simulink model "padTracking"  (R2014a)
settings: Solver=FixedStepDiscrete  StartTime=0.0  StopTime=inf  RelTol=1e-3
undefined symbols (not defined in the file or in its folder): fdesignblkfcn, gcbh
libraries: simulink x6, visionstatistics x3, visiontextngfix x2, embdlinuxlib x2
settings Model: SimulationMode=external  ExtModeTrigDuration=100  Creator=omcaree  LastModifiedBy=jsustare
settings OptimizationCC: OptimizeModelRefInitCode=on  LifeSpan=1
settings DebuggingCC: UnderspecifiedInitializationDetection=Classic  SolverPrmCheckMsg=none
settings HardwareCC: ProdLargestAtomicInteger=Long  ProdLargestAtomicFloat=Double  ProdEndianess=LittleEndian  ProdHWDeviceType=ARM Compatible->ARM Cortex
settings RTWCC: SystemTargetFile=realtime.tlc  GenerateMakefile=off  TemplateMakefile=realtime.tmf  Description=Run on Target Hardware  RTWVerbose=off  ProcessScript=realtime_make_rtw_hook
settings STFCustomTargetCC: TargetLibSuffix=.a  GenerateSampleERTMain=on  ConcurrentExecutionCompliant=off  GeneratePreprocessorConditionals=Use local settings  ERTCustomFileBanners=on  SupportNonInlinedSFcns=off  SupportVariableSizeSignals=on  MATLABClassNameForMDSCustomization=Simulink.SoftwareTarget.ERTCustomization  GRTInterface=off  SystemTargetFile=realtime.tlc
settings ERTTargetCC: CombineOutputUpdateFcns=off  SupportContinuousTime=on  SupportVariableSizeSignals=on  ExtMode=on  ExtModeMexArgs='169.254.0.31' 0 17725  ERTSrcFileBannerTemplate=realtime_code_template.cgt  ERTHdrFileBannerTemplate=realtime_code_template.cgt  ERTDataSrcFileTemplate=realtime_code_template.cgt  ERTDataHdrFileTemplate=realtime_code_template.cgt  ERTCustomFileTemplate=realtime_file_process.tlc

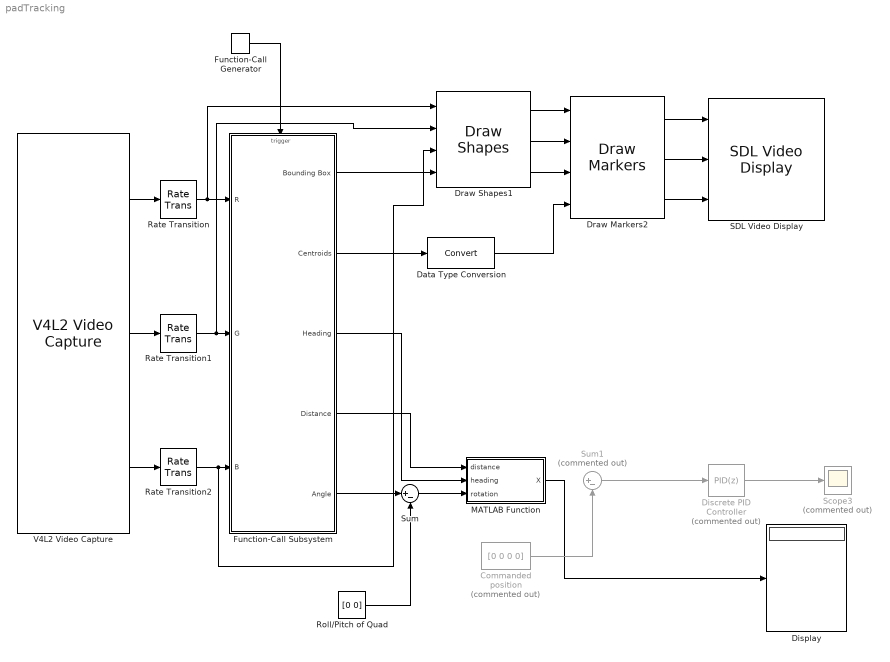
== system padTracking ==
  Commanded position : Constant  Commented=on  Value=[0 0 0 0]
  Data Type Conversion : DataTypeConversion
  Discrete PID Controller : simulink/Continuous/PID Controller  Commented=on  Controller=PID  TimeDomain=Discrete-time  SampleTime=-1  IntegratorMethod=Forward Euler  FilterMethod=Forward Euler  Form=Parallel  P=[1 1 1 1]  I=[0 0 0 0]  D=[0 0 0 0]  N=100  InitialConditionSource=internal  InitialConditionForIntegrator=0  InitialConditionForFilter=0  ExternalReset=none  LimitOutput=off  UpperSaturationLimit=inf  LowerSaturationLimit=-inf  LinearizeAsGain=off  AntiWindupMode=none  Kb=1  TrackingMode=off  Kt=1  PParamMin=[]  PParamMax=[]  IParamMin=[]  IParamMax=[]  DParamMin=[]  DParamMax=[]  NParamMin=[]  NParamMax=[]  KbParamMin=[]  KbParamMax=[]  KtParamMin=[]  KtParamMax=[]  POutMin=[]  POutMax=[]  IOutMin=[]  IOutMax=[]  DOutMin=[]  DOutMax=[]  NOutMin=[]  NOutMax=[]  KbOutMin=[]  KbOutMax=[]  KtOutMin=[]  KtOutMax=[]  IntegratorOutMin=[]  IntegratorOutMax=[]  FilterOutMin=[]  FilterOutMax=[]  SumOutMin=[]  SumOutMax=[]  SumI1OutMin=[]  SumI1OutMax=[]  SumI2OutMin=[]  SumI2OutMax=[]  SumI3OutMin=[]  SumI3OutMax=[]  SumDOutMin=[]  SumDOutMax=[]  SaturationOutMin=[]  SaturationOutMax=[]  IntegratorContinuousStateAttributes=''  IntegratorStateMustResolveToSignalObject=off  IntegratorRTWStateStorageClass=Auto  FilterContinuousStateAttributes=''  FilterStateMustResolveToSignalObject=off  FilterRTWStateStorageClass=Auto
  Display : Display
  Draw Markers2 : visiontextngfix/Draw Markers  shape=X-mark  size=3  fill=off  fillClrSource=Specify via dialog  display=User-specified value  intensity=200  color=[0 255 0; 255 0 0; 255 255 255]  opacity=0.6  viewport=Entire image  antialiasing=off  inType=Obsolete  imagePorts=Separate color signals  prodOutputMode=Binary point scaling  prodOutputWordLength=32  prodOutputFracLength=14  memoryMode=Specify word length  memoryWordLength=16  memoryFracLength=15  roundingMode=Floor  overflowMode=off
  Draw Shapes1 : visiontextngfix/Draw Shapes  shape=Rectangles  fill=off  lineWidth=1  fillClrSource=Specify via dialog  display=User-specified value  intensity=200  color=[255 0 0]  opacity=0.6  viewport=Entire image  antialiasing=off  inType=Obsolete  imagePorts=Separate color signals  prodOutputMode=Binary point scaling  prodOutputWordLength=32  prodOutputFracLength=14  memoryMode=Specify word length  memoryWordLength=16  memoryFracLength=15  roundingMode=Floor  overflowMode=off
  Function-Call Generator : simulink/Ports & Subsystems/Function-Call Generator  sample_time=3/30  numberOfIterations=1
  Function-Call Subsystem : Subsystem  TreatAsAtomicUnit=on
  MATLAB Function : MATLAB Function  TreatAsAtomicUnit=on
  Rate Transition : RateTransition  Deterministic=off
  Rate Transition1 : RateTransition  Deterministic=off
  Rate Transition2 : RateTransition  Deterministic=off
  Roll/Pitch of Quad : Constant  Value=[0 0]
  SDL Video Display : embdlinuxlib/SDL Video Display  pixelFormat=RGB  pixelOrder=Planar  rowMajor=on  blockPlatform=Raspberry Pi
  Scope3 : Scope  Commented=on
      settings: YMin=-0.05  YMax=0.65  SaveName=ScopeData3
  Sum : Sum  Inputs=|+-
  Sum1 : Sum  Commented=on  Inputs=|+-
  V4L2 Video Capture : embdlinuxlib/V4L2 Video Capture  m_devName='/dev/video0'  roi=[0, 0, 640, 480]  imSizeSelection=320x240  imSize=[640, 480]  pixelFormat=RGB  pixelOrder=Planar  sampleTime=1/30  simOutput=Colorbars  blockPlatform=Raspberry Pi
  wires:
  V4L2 Video Capture/3 -> Rate Transition2/1
  V4L2 Video Capture/1 -> Rate Transition/1
  V4L2 Video Capture/2 -> Rate Transition1/1
  Function-Call Generator/1 -> Function-Call Subsystem/Trigger
  Function-Call Subsystem/1(Bounding Box) -> Draw Shapes1/4
  Rate Transition/1 -> Draw Shapes1/1, Function-Call Subsystem/1(R)
  Rate Transition1/1 -> Draw Shapes1/2, Function-Call Subsystem/2(G)
  Rate Transition2/1 -> Draw Shapes1/3, Function-Call Subsystem/3(B)
  Data Type Conversion/1 -> Draw Markers2/4
  Function-Call Subsystem/2(Centroids) -> Data Type Conversion/1
  Function-Call Subsystem/4("Distance ") -> MATLAB Function/1(distance)
  Function-Call Subsystem/5(Angle) -> Sum/1
  Sum/1 -> MATLAB Function/3(rotation)
  Roll/Pitch of Quad/1 -> Sum/2
  MATLAB Function/1(X) -> Display/1
  Commanded position/1 -> Sum1/2
  Sum1/1 -> Discrete PID Controller/1
  Discrete PID Controller/1 -> Scope3/1
  Draw Markers2/2 -> SDL Video Display/2
  Draw Markers2/3 -> SDL Video Display/3
  Draw Markers2/1 -> SDL Video Display/1
  Draw Shapes1/3 -> Draw Markers2/3
  Draw Shapes1/2 -> Draw Markers2/2
  Draw Shapes1/1 -> Draw Markers2/1
  Function-Call Subsystem/3(Heading) -> MATLAB Function/2(heading)

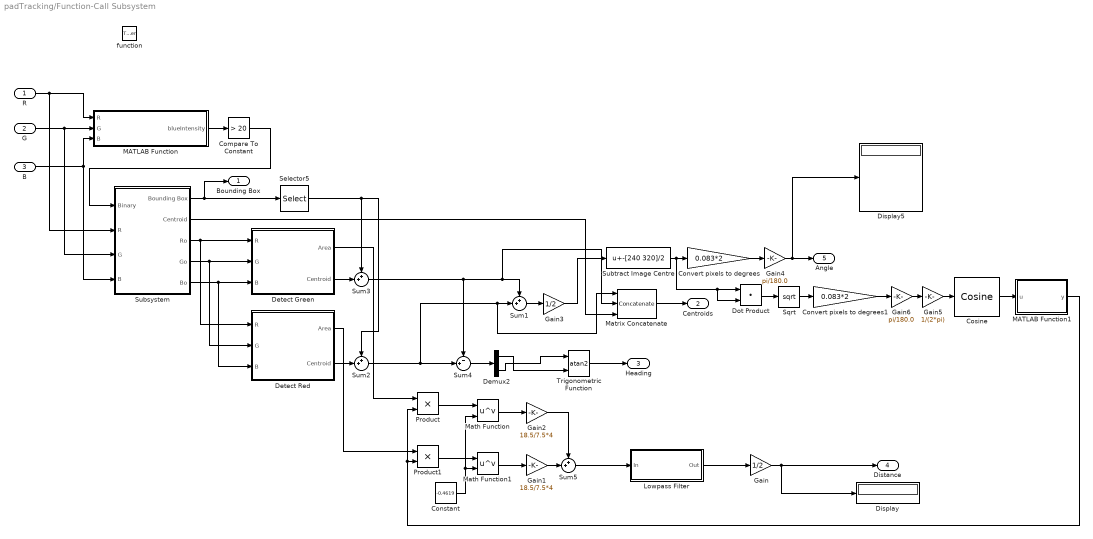
== system padTracking/Function-Call Subsystem ==
  R : Inport
  G : Inport  Port=2
  B : Inport  Port=3
  function : TriggerPort  TriggerType=function-call
  Compare To Constant : simulink/Logic and Bit Operations/Compare To Constant  relop=>  const=20  OutDataTypeStr=boolean
  Constant : Constant  Value=-0.4619
  Convert pixels to degrees : Gain  Gain=0.083*2
  Convert pixels to degrees1 : Gain  Gain=0.083*2
  Cosine : simulink/Lookup Tables/Cosine  Formula=cos(2*pi*u)  NumDataPoints=(2^5)+1  OutputWordLength=16  InternalRulePriority=Speed
  Demux2 : Demux  Outputs=2
  Detect Green : Subsystem
  Detect Red : Subsystem
  Display : Display
  Display5 : Display
  Dot Product : DotProduct  InputSameDT=on  OutDataTypeStr=Inherit: Inherit via internal rule
  Gain : Gain  Gain=1/2
  Gain1 : Gain  Gain=18.5/7.5*4
  Gain2 : Gain  Gain=18.5/7.5*4
  Gain3 : Gain  Gain=1/2
  Gain4 : Gain  Gain=pi/180.0
  Gain5 : Gain  Gain=1/(2*pi)
  Gain6 : Gain  Gain=pi/180.0
  Lowpass Filter : Subsystem  DialogController=fdesignblkfcn  InitFcn=fdesignblkfcn(gcbh, {'InitFcn'});  mask(Lowpass Filter){}
      mask help: Design a lowpass filter
      settings: CopyFcn=fdesignblkfcn(gcbh, {'CopyFcn'});
      mask Help: helpview(mapfilelocation('dsp'), 'dsplowpassfilter');
      mask Display: disp('Lowpass')
  MATLAB Function : MATLAB Function  TreatAsAtomicUnit=on
  MATLAB Function1 : MATLAB Function  TreatAsAtomicUnit=on
  Math Function : Math  Operator=pow  SaturateOnIntegerOverflow=on
  Math Function1 : Math  Operator=pow  SaturateOnIntegerOverflow=on
  Matrix Concatenate : Concatenate  NumInputs=3  Mode=Multidimensional array
  Product : Product
  Product1 : Product
  Selector5 : Selector  InputPortWidth=4  Indices=[1 2]
  Sqrt : Sqrt  SaturateOnIntegerOverflow=on
  Subsystem : Subsystem
  Subtract Image Centre : Bias  Bias=-[240 320]/2
  Sum{1..3,5} (4 alike) : Sum  Inputs=++|
  Sum4 : Sum  Inputs=-+|
  Trigonometric Function : Trigonometry  Operator=atan2
  Bounding Box : Outport
  Centroids : Outport  Port=2
  Heading : Outport  Port=3
  "Distance " : Outport  Port=4
  Angle : Outport  Port=5
  wires:
  G/1 -> MATLAB Function/2(G), Subsystem/3(G)
  R/1 -> MATLAB Function/1(R), Subsystem/2(R)
  MATLAB Function/1(blueIntensity) -> Compare To Constant/1
  Compare To Constant/1 -> Subsystem/1(Binary)
  B/1 -> Subsystem/4(B), MATLAB Function/3(B)
  Selector5/1 -> Sum3/1, Sum2/1
  Sum2/1 -> Matrix Concatenate/1, Sum1/2, Sum4/2
  Sum4/1 -> Demux2/1
  Math Function1/1 -> Gain1/1
  Math Function/1 -> Gain2/1
  Constant/1 -> Math Function/2, Math Function1/2
  Demux2/2 -> Trigonometric Function/1
  Demux2/1 -> Trigonometric Function/2
  Detect Green/1(Area) -> Product/1
  Detect Green/2(Centroid) -> Sum3/2
  Detect Red/1(Area) -> Product1/1
  Detect Red/2(Centroid) -> Sum2/2
  Subsystem/3(Ro) -> Detect Red/1(R), Detect Green/1(R)
  Subsystem/5(Bo) -> Detect Red/3(B), Detect Green/3(B)
  Subsystem/4(Go) -> Detect Red/2(G), Detect Green/2(G)
  Subsystem/1(Bounding Box) -> Selector5/1, Bounding Box/1
  Trigonometric Function/1 -> Heading/1
  Gain/1 -> "Distance "/1, Display/1
  Sum1/1 -> Gain3/1
  Gain3/1 -> Subtract Image Centre/1
  Sum3/1 -> Matrix Concatenate/2, Sum1/1, Sum4/1
  Gain2/1 -> Sum5/1
  Gain1/1 -> Sum5/2
  Subtract Image Centre/1 -> Dot Product/2, Dot Product/1, Convert pixels to degrees/1
  Convert pixels to degrees/1 -> Gain4/1
  Gain4/1 -> Display5/1, Angle/1
  Matrix Concatenate/1 -> Centroids/1
  Subsystem/2(Centroid) -> Matrix Concatenate/3
  Lowpass Filter/1(Out) -> Gain/1
  Gain5/1 -> Cosine/1
  Convert pixels to degrees1/1 -> Gain6/1
  Gain6/1 -> Gain5/1
  Dot Product/1 -> Sqrt/1
  Sqrt/1 -> Convert pixels to degrees1/1
  Sum5/1 -> Lowpass Filter/1(In)
  Product/1 -> Math Function/1
  Product1/1 -> Math Function1/1
  MATLAB Function1/1(y) -> Product1/2, Product/2
  Cosine/1 -> MATLAB Function1/1(u)

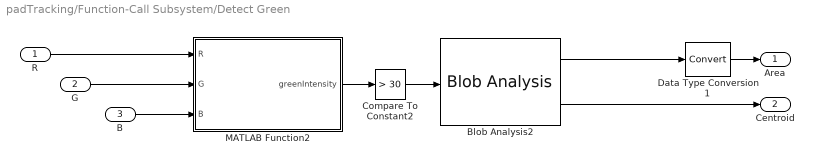
== system padTracking/Function-Call Subsystem/Detect Green ==
  R : Inport
  G : Inport  Port=2
  B : Inport  Port=3
  Blob Analysis2 : visionstatistics/Blob Analysis  Tag=vipblks_row_conv  area=on  centroid=on  bBox=off  majorAxis=off  minorAxis=off  angle=off  eccentricity=off  equivDiameterSq=off  extent=off  perimeter=off  maxBlobs=1  warnIfNumBlobsExceeded=on  isCount=off  useMinArea=off  minArea=0  useMaxArea=off  maxArea=intmax('uint32')  excludeBorderBlob=off  outDT=double  isOutVarDim=off  isFill=on  fillValues=-1  conn=8  isLabel=off  outputMode=Binary point scaling  outputWordLength=32  outputFracLength=16  firstCoeffMode=Binary point scaling  firstCoeffWordLength=16  firstCoeffFracLength=14  secondCoeffMode=Binary point scaling  secondCoeffWordLength=32  secondCoeffFracLength=16  accumMode=Binary point scaling  accumWordLength=32  accumFracLength=0  prodOutputMode=Binary point scaling  prodOutputWordLength=32  prodOutputFracLength=16  roundingMode=Floor  overflowMode=off
  Compare To Constant2 : simulink/Logic and Bit Operations/Compare To Constant  relop=>  const=30  OutDataTypeStr=boolean
  Data Type Conversion1 : DataTypeConversion
  MATLAB Function2 : MATLAB Function  TreatAsAtomicUnit=on
  Area : Outport
  Centroid : Outport  Port=2
  wires:
  B/1 -> MATLAB Function2/3(B)
  R/1 -> MATLAB Function2/1(R)
  G/1 -> MATLAB Function2/2(G)
  MATLAB Function2/1(greenIntensity) -> Compare To Constant2/1
  Compare To Constant2/1 -> Blob Analysis2/1
  Blob Analysis2/2 -> Centroid/1
  Blob Analysis2/1 -> Data Type Conversion1/1
  Data Type Conversion1/1 -> Area/1

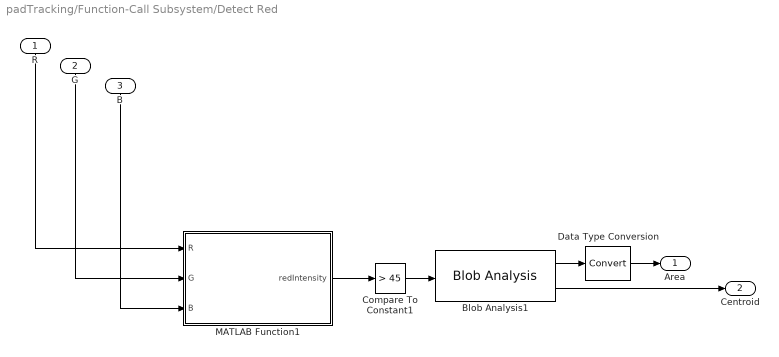
== system padTracking/Function-Call Subsystem/Detect Red ==
  R : Inport
  G : Inport  Port=2
  B : Inport  Port=3
  Blob Analysis1 : visionstatistics/Blob Analysis  Tag=vipblks_row_conv  area=on  centroid=on  bBox=off  majorAxis=off  minorAxis=off  angle=off  eccentricity=off  equivDiameterSq=off  extent=off  perimeter=off  maxBlobs=1  warnIfNumBlobsExceeded=on  isCount=off  useMinArea=off  minArea=0  useMaxArea=off  maxArea=intmax('uint32')  excludeBorderBlob=off  outDT=double  isOutVarDim=off  isFill=on  fillValues=-1  conn=8  isLabel=off  outputMode=Binary point scaling  outputWordLength=32  outputFracLength=16  firstCoeffMode=Binary point scaling  firstCoeffWordLength=16  firstCoeffFracLength=14  secondCoeffMode=Binary point scaling  secondCoeffWordLength=32  secondCoeffFracLength=16  accumMode=Binary point scaling  accumWordLength=32  accumFracLength=0  prodOutputMode=Binary point scaling  prodOutputWordLength=32  prodOutputFracLength=16  roundingMode=Floor  overflowMode=off
  Compare To Constant1 : simulink/Logic and Bit Operations/Compare To Constant  relop=>  const=45  OutDataTypeStr=boolean
  Data Type Conversion : DataTypeConversion
  MATLAB Function1 : MATLAB Function  TreatAsAtomicUnit=on
  Area : Outport
  Centroid : Outport  Port=2
  wires:
  R/1 -> MATLAB Function1/1(R)
  B/1 -> MATLAB Function1/3(B)
  G/1 -> MATLAB Function1/2(G)
  MATLAB Function1/1(redIntensity) -> Compare To Constant1/1
  Compare To Constant1/1 -> Blob Analysis1/1
  Blob Analysis1/2 -> Centroid/1
  Blob Analysis1/1 -> Data Type Conversion/1
  Data Type Conversion/1 -> Area/1

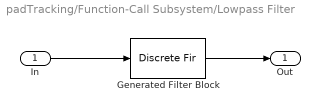
== system padTracking/Function-Call Subsystem/Lowpass Filter ==
  In : Inport
  Generated Filter Block : DiscreteFir  Tag=BlockMethodSubSystem  Coefficients=[0.011901508381575016 0.02908797826733928 0.0025913585662860131 -0.068996275507793012 -0.050025679925086837 0.16540100530640869 0.41332778671981452 0.41332778671981452 0.16540100530640869 -0.050025679925086837 -0.068996275507793012 0.0025913585662860131 0.02908797826733928 0.011901508381575016]  InputProcessing=Columns as channels (frame based)
  Out : Outport
  wires:
  In/1 -> Generated Filter Block/1
  Generated Filter Block/1 -> Out/1

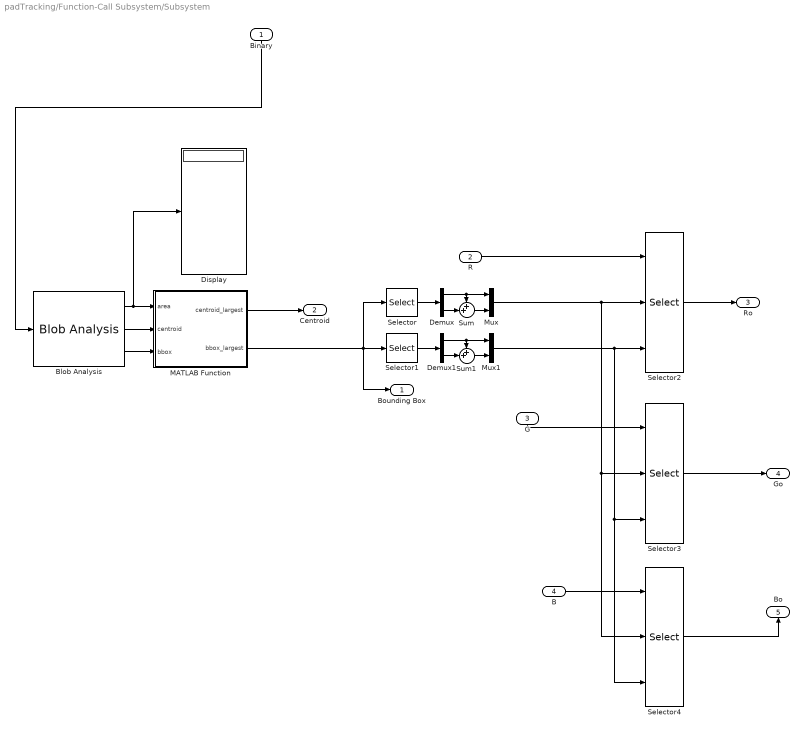
== system padTracking/Function-Call Subsystem/Subsystem ==
  Binary : Inport
  R : Inport  Port=2
  G : Inport  Port=3
  B : Inport  Port=4
  Blob Analysis : visionstatistics/Blob Analysis  Tag=vipblks_row_conv  area=on  centroid=on  bBox=on  majorAxis=off  minorAxis=off  angle=off  eccentricity=off  equivDiameterSq=off  extent=off  perimeter=off  maxBlobs=16  warnIfNumBlobsExceeded=on  isCount=off  useMinArea=on  minArea=64  useMaxArea=off  maxArea=intmax('uint32')  excludeBorderBlob=on  outDT=double  isOutVarDim=off  isFill=on  fillValues=-1  conn=8  isLabel=off  outputMode=Binary point scaling  outputWordLength=32  outputFracLength=16  firstCoeffMode=Binary point scaling  firstCoeffWordLength=16  firstCoeffFracLength=14  secondCoeffMode=Binary point scaling  secondCoeffWordLength=32  secondCoeffFracLength=16  accumMode=Binary point scaling  accumWordLength=32  accumFracLength=0  prodOutputMode=Binary point scaling  prodOutputWordLength=32  prodOutputFracLength=16  roundingMode=Floor  overflowMode=off
  Demux : Demux  Outputs=2
  Demux1 : Demux  Outputs=2
  Display : Display
  MATLAB Function : MATLAB Function  TreatAsAtomicUnit=on
  Mux : Mux  Inputs=2
  Mux1 : Mux  Inputs=2
  Selector : Selector  InputPortWidth=4  Indices=[2 4]
  Selector1 : Selector  InputPortWidth=4  Indices=[1 3]
  Selector2 : Selector  NumberOfDimensions=2  InputPortWidth=4  IndexOptions=Starting and ending indices (port),Starting and ending indices (port)  Indices=[2 4],1  OutputSizes=1,1
  Selector3 : Selector  NumberOfDimensions=2  InputPortWidth=4  IndexOptions=Starting and ending indices (port),Starting and ending indices (port)  Indices=[2 4],1  OutputSizes=1,1
  Selector4 : Selector  NumberOfDimensions=2  InputPortWidth=4  IndexOptions=Starting and ending indices (port),Starting and ending indices (port)  Indices=[2 4],1  OutputSizes=1,1
  Sum : Sum  Inputs=++|
  Sum1 : Sum  Inputs=++|
  Bounding Box : Outport
  Centroid : Outport  Port=2
  Ro : Outport  Port=3
  Go : Outport  Port=4
  Bo : Outport  Port=5
  wires:
  G/1 -> Selector3/1
  R/1 -> Selector2/1
  Binary/1 -> Blob Analysis/1
  B/1 -> Selector4/1
  Selector/1 -> Demux/1
  Selector1/1 -> Demux1/1
  Demux/2 -> Sum/2
  Demux/1 -> Mux/1, Sum/1
  Sum/1 -> Mux/2
  Demux1/1 -> Sum1/1, Mux1/1
  Sum1/1 -> Mux1/2
  Demux1/2 -> Sum1/2
  Selector2/1 -> Ro/1
  Selector3/1 -> Go/1
  Selector4/1 -> Bo/1
  Blob Analysis/3 -> MATLAB Function/3(bbox)
  Blob Analysis/1 -> MATLAB Function/1(area), Display/1
  Mux/1 -> Selector4/2, Selector3/2, Selector2/2
  Mux1/1 -> Selector4/3, Selector3/3, Selector2/3
  MATLAB Function/2(bbox_largest) -> Bounding Box/1, Selector1/1, Selector/1
  MATLAB Function/1(centroid_largest) -> Centroid/1
  Blob Analysis/2 -> MATLAB Function/2(centroid)

== matlab function padTracking/Function-Call Subsystem/Detect Red/MATLAB Function1 ==
  data: R input; redIntensity output size=[320 240]; G input; B input
function redIntensity = fcn(R,G,B)
%#codegen
redIntensity = R - G/2 - B/2;

== matlab function padTracking/Function-Call Subsystem/MATLAB Function ==
  data: R input; blueIntensity output; G input; B input
function blueIntensity = fcn(R,G,B)
%#codegen

blueIntensity = B - R/2 - G/2;

== matlab function padTracking/Function-Call Subsystem/Detect Green/MATLAB Function2 ==
  data: R input; greenIntensity output size=[320 240]; G input; B input
function greenIntensity = fcn(R,G,B)
%#codegen

greenIntensity = G - R/2 - B/2;

== matlab function padTracking/MATLAB Function ==
  data: distance input; X output; heading input; rotation input
function X  = fcn(distance,heading,rotation)
%#codegen

X_local = -distance*[sin(rotation(1)); -sin(rotation(2))];
R = [cos(-heading) sin(-heading); -sin(-heading) cos(-heading)];
X = [R*X_local;distance;heading];

== matlab function padTracking/Function-Call Subsystem/Subsystem/MATLAB Function ==
  data: centroid_largest output; area input; centroid input; bbox_largest output; bbox input
function [centroid_largest, bbox_largest] = selectLargest(area, centroid, bbox)
%#codegen

[y, i] = max(area);
bbox_largest = bbox(i,:);
centroid_largest = centroid(i,:);

== matlab function padTracking/Function-Call Subsystem/MATLAB Function1 ==
  data: u input; y output
function y = fcn(u)
%#codegen

y = u^2;
